simulink model "downlink_8c4t"  (Simulink 8.7)
settings: Solver=VariableStepDiscrete  StartTime=0.0  StopTime=20000  RelTol=1e-3
PreLoadFcn:
  | % Run the setup script when the model is opened
  | setup_downlink_8c4t;
InitFcn:
  | % Run the setup script again just before the
  | % model is run, so that any updates made
  | % after opening are applied.
  | 
  | setup_downlink_8c4t;
  | 
  | 
  | %% DSPBuilder Start
  | alt_dspbuilder_update_model(bdroot)
  | %% DSPBuilder End
values from neighbouring files (symbols this model uses):
  LUTS =     [downlink_8c4t_luts2.mat]
undefined symbols (not defined in the file or in its folder): DUC_LINEUP_param, value
libraries: DSPBAModelBus x44, DSPBABase x9, pipereg_lib x6, blind_cfr_lib x4, hduc_lib x4, dpd_lib x4, simulink x2, mixer_lib x2, lduc_lib x2, summer_4c4t_lib x2, DSPBAPrim x1
(part 1 of 2)
Description:
  | DSP Builder Advanced Template for Template Design implementing ModelIP designs
settings Model: Creator=mjervis  LastModifiedBy=5g
settings DataIOCC: SignalLoggingSaveFormat=ModelDataLogs
settings OptimizationCC: ExpressionDepthLimit=2147483647
settings DebuggingCC: SolverPrmCheckMsg=warning  InheritedTsInSrcMsg=none  IntegerOverflowMsg=none  FcnCallInpInsideContextMsg=UseLocalSettings  StateNameClashWarn=warning  IntegerSaturationMsg=none
settings GRTTargetCC: CombineOutputUpdateFcns=off  GRTInterface=on
settings ConfigComp: CovSFcnEnable=off

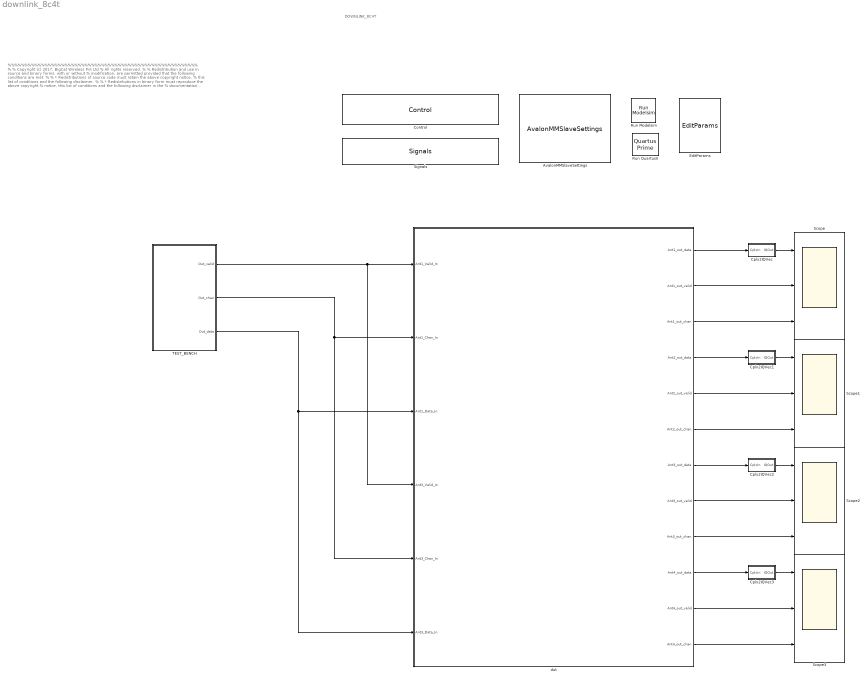
== system downlink_8c4t ==
  note: %%%%%%%%%%%%%%%%%%%%%%%%%%%%%%%%%%%%%%%%%%%%%%%%%%%%%%%%%
      | %
      | % Copyright (c) 2017, BigCat Wireless Pvt Ltd
      | % All rights reserved.
      | %
      | % Redistribution and use in source and binary forms, with or without
      | % modification, are permitted provided that the following conditions are met:
      | %
      | % * Redistributions of source code must retain the above copyright notice,
      | % this list of conditions and the following disclaimer.
      | %
      | % * Redistributions in binary form must reproduce the above copyright
      | % notice, this list of conditions and the following disclaimer in the
      | % documentation and/or other materials provided with the distribution.
      | %
      | % * Neither the name of the copyright holder nor the names of its contributors
      | % may be used to endorse or promote products derived from this software
      | % without specific prior written permission.
      | %
      | %
      | %
      | % THIS SOFTWARE IS PROVIDED BY THE COPYRIGHT HOLDERS AND CONTRIBUTORS "AS IS"
      | % AND ANY EXPRESS OR IMPLIED WARRANTIES, INCLUDING, BUT NOT LIMITED TO, THE
      | % IMPLIED WARRANTIES OF MERCHANTABILITY AND FITNESS FOR A PARTICULAR PURPOSE ARE
      | % DISCLAIMED. IN NO EVENT SHALL THE COPYRIGHT HOLDER OR CONTRIBUTORS BE LIABLE
      | % FOR ANY DIRECT, INDIRECT, INCIDENTAL, SPECIAL, EXEMPLARY, OR CONSEQUENTIAL
      | % DAMAGES (INCLUDING, BUT NOT LIMITED TO, PROCUREMENT OF SUBSTITUTE GOODS OR
      | % SERVICES; LOSS OF USE, DATA, OR PROFITS; OR BUSINESS INTERRUPTION) HOWEVER
      | % CAUSED AND ON ANY THEORY OF LIABILITY, WHETHER IN CONTRACT, STRICT LIABILITY,
      | % OR TORT (INCLUDING NEGLIGENCE OR OTHERWISE) ARISING IN ANY WAY OUT OF THE USE
      | % OF THIS SOFTWARE, EVEN IF ADVISED OF THE POSSIBILITY OF SUCH DAMAGE.
      | %
      | %%%%%%%%%%%%%%%%%%%%%%%%%%%%%%%%%%%%%%%%%%%%%%%%%%%%%%%%%%
  note: DOWNLINK_8C4T
  AvalonMMSlaveSettings : DSPBABase/AvalonMMSlaveSettings
  Control : DSPBABase/Control  generate=on  language=VHDL  destination=./rtl  destination_gui=./rtl  make_full_path=off  path_is_relative=on  autotestbench=off  signaldepth=2  coveragetestbench=off  logs=off  spacewidth=2  spacenum=1  addrwidth=13  datawidth=32  dataendian=Big Endian  hierarchicalnames=off  ramThresholdBits=-1  distRamThresholdBits=-1  mlabThresholdBits=-1  hardMultiplierThresholdLuts=-1  version=20090407  errorOnChanMismatch=1  errorOnGPIOMismatch=0  importModelsimResults=0  cycleAccurate=off  reinterpretCastMult=off  paramFile=downlink_8c4t_params.xml
  Cplx2IQVec : Subsystem
  Cplx2IQVec1 : Subsystem
  Cplx2IQVec2 : Subsystem
  Cplx2IQVec3 : Subsystem
  EditParams : DSPBABase/EditParams  version=20090407
  Run Modelsim : DSPBABase/Run Modelsim  version=20090407
  "Run QuartusII " : DSPBABase/Quartus Prime  version=20090407
  Scope{,1..3} (4 alike) : Scope  NumInputPorts=3
  Signals : DSPBABase/Signals  clk=clk  freq=DUC_LINEUP_param.ClockRate  margin=DUC_LINEUP_param.ClockMargin  rst=areset  rstactive=High  bus=bus  enbusclock=on  busfreq=61.44  bussync=on  version=20090407
  TEST_BENCH : Subsystem
  dut : Subsystem
  wires:
  TEST_BENCH/2(Out_chan) -> dut/5(Ant3_Chan_In), dut/2(Ant1_Chan_In)
  TEST_BENCH/3(Out_data) -> dut/6(Ant3_Data_In), dut/3(Ant1_Data_In)
  TEST_BENCH/1(Out_valid) -> dut/4(Ant3_Valid_In), dut/1(Ant1_Valid_In)
  dut/1(Ant1_out_data) -> Cplx2IQVec/1(CplxIn)
  dut/2(Ant1_out_valid) -> Scope/2
  dut/3(Ant1_out_chan) -> Scope/3
  dut/4(Ant2_out_data) -> Cplx2IQVec1/1(CplxIn)
  dut/5(Ant2_out_valid) -> Scope1/2
  dut/6(Ant2_out_chan) -> Scope1/3
  dut/7(Ant3_out_data) -> Cplx2IQVec2/1(CplxIn)
  dut/8(Ant3_out_valid) -> Scope2/2
  dut/9(Ant3_out_chan) -> Scope2/3
  dut/10(Ant4_out_data) -> Cplx2IQVec3/1(CplxIn)
  dut/11(Ant4_out_valid) -> Scope3/2
  dut/12(Ant4_out_chan) -> Scope3/3
  Cplx2IQVec/1(IQOut) -> Scope/1
  Cplx2IQVec1/1(IQOut) -> Scope1/1
  Cplx2IQVec2/1(IQOut) -> Scope2/1
  Cplx2IQVec3/1(IQOut) -> Scope3/1

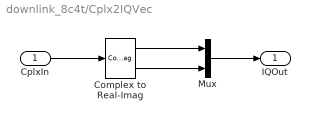
== system downlink_8c4t/Cplx2IQVec ==
  CplxIn : Inport
  Complex to Real-Imag : ComplexToRealImag
  Mux : Mux  Inputs=2
  IQOut : Outport
  wires:
  Complex to Real-Imag/1 -> Mux/1
  Mux/1 -> IQOut/1
  Complex to Real-Imag/2 -> Mux/2
  CplxIn/1 -> Complex to Real-Imag/1

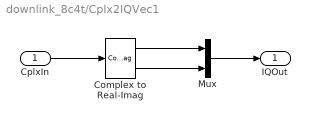
== system downlink_8c4t/Cplx2IQVec1 ==
  CplxIn : Inport
  Complex to Real-Imag : ComplexToRealImag
  Mux : Mux  Inputs=2
  IQOut : Outport
  wires:
  CplxIn/1 -> Complex to Real-Imag/1
  Complex to Real-Imag/2 -> Mux/2
  Mux/1 -> IQOut/1
  Complex to Real-Imag/1 -> Mux/1

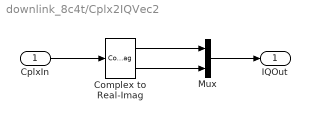
== system downlink_8c4t/Cplx2IQVec2 ==
  CplxIn : Inport
  Complex to Real-Imag : ComplexToRealImag
  Mux : Mux  Inputs=2
  IQOut : Outport
  wires:
  Complex to Real-Imag/1 -> Mux/1
  Mux/1 -> IQOut/1
  Complex to Real-Imag/2 -> Mux/2
  CplxIn/1 -> Complex to Real-Imag/1

== system downlink_8c4t/Cplx2IQVec3 ==
  CplxIn : Inport
  Complex to Real-Imag : ComplexToRealImag
  Mux : Mux  Inputs=2
  IQOut : Outport
  wires:
  CplxIn/1 -> Complex to Real-Imag/1
  Complex to Real-Imag/2 -> Mux/2
  Mux/1 -> IQOut/1
  Complex to Real-Imag/1 -> Mux/1

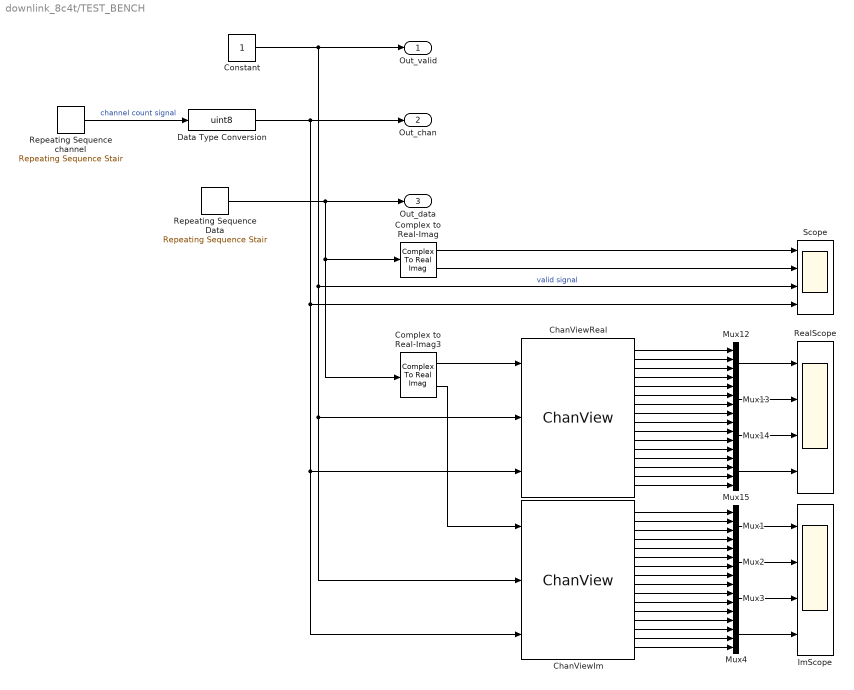
== system downlink_8c4t/TEST_BENCH ==
  ChanViewIm : DSPBABase/ChanView  nchans=16  chan_vector=[0:15]  outsvalid=off  latency=1  version=20090407
  ChanViewReal : DSPBABase/ChanView  nchans=16  chan_vector=[0:15]  outsvalid=off  latency=1  version=20090407
  Complex to Real-Imag : ComplexToRealImag
  Complex to Real-Imag3 : ComplexToRealImag
  Constant : Constant  OutDataTypeStr=boolean  SampleTime=1
  Data Type Conversion : DataTypeConversion  OutDataTypeStr=uint8
  ImScope : Scope  NumInputPorts=4
  Mux{1..4,12..15} (8 alike) : Mux
  RealScope : Scope  NumInputPorts=4
  Repeating Sequence Data : simulink/Sources/Repeating Sequence Stair  OutValues=DUC_LINEUP_param.inputdata  tsamp=1  OutMin=[]  OutMax=[]  OutDataTypeStr=fixdt(1,16,15)  OutputDataTypeScalingMode=Specify via dialog  OutDataType=fixdt(1,16,15)  ConRadixGroup=Best Precision: Vector-wise  OutScaling=[]
  Repeating Sequence channel : simulink/Sources/Repeating Sequence Stair  OutValues=[0:15].'  tsamp=1  OutMin=[]  OutMax=[]  OutDataTypeStr=uint8  OutputDataTypeScalingMode=uint8  OutDataType=fixdt(1,16)  ConRadixGroup=Best Precision: Vector-wise  OutScaling=[]
  Scope : Scope  NumInputPorts=4
  Out_valid : Outport
  Out_chan : Outport  Port=2
  Out_data : Outport  Port=3
  wires:
  Repeating Sequence Data/1 -> Out_data/1, Complex to Real-Imag/1, Complex to Real-Imag3/1
  Complex to Real-Imag/1 -> Scope/1
  Constant/1 -> Out_valid/1, ChanViewIm/2, ChanViewReal/2, Scope/3  "valid signal"
  Repeating Sequence channel/1 -> Data Type Conversion/1  "channel count signal"
  Complex to Real-Imag/2 -> Scope/2
  Mux12/1 -> RealScope/1
  Mux13/1 -> RealScope/2
  Mux14/1 -> RealScope/3
  Mux15/1 -> RealScope/4
  Complex to Real-Imag3/1 -> ChanViewReal/1
  Complex to Real-Imag3/2 -> ChanViewIm/1
  ChanViewReal/2 -> Mux12/2
  ChanViewReal/4 -> Mux12/4
  ChanViewReal/1 -> Mux12/1
  ChanViewReal/3 -> Mux12/3
  ChanViewReal/8 -> Mux13/4
  ChanViewReal/5 -> Mux13/1
  ChanViewReal/6 -> Mux13/2
  ChanViewReal/7 -> Mux13/3
  ChanViewReal/12 -> Mux14/4
  ChanViewReal/9 -> Mux14/1
  ChanViewReal/11 -> Mux14/3
  ChanViewReal/10 -> Mux14/2
  ChanViewReal/15 -> Mux15/3
  ChanViewReal/13 -> Mux15/1
  ChanViewReal/16 -> Mux15/4
  ChanViewReal/14 -> Mux15/2
  Mux1/1 -> ImScope/1
  Mux2/1 -> ImScope/2
  Mux3/1 -> ImScope/3
  Mux4/1 -> ImScope/4
  ChanViewIm/2 -> Mux1/2
  ChanViewIm/4 -> Mux1/4
  ChanViewIm/1 -> Mux1/1
  ChanViewIm/3 -> Mux1/3
  ChanViewIm/8 -> Mux2/4
  ChanViewIm/5 -> Mux2/1
  ChanViewIm/6 -> Mux2/2
  ChanViewIm/7 -> Mux2/3
  ChanViewIm/12 -> Mux3/4
  ChanViewIm/9 -> Mux3/1
  ChanViewIm/11 -> Mux3/3
  ChanViewIm/10 -> Mux3/2
  ChanViewIm/15 -> Mux4/3
  ChanViewIm/13 -> Mux4/1
  ChanViewIm/16 -> Mux4/4
  ChanViewIm/14 -> Mux4/2
  Data Type Conversion/1 -> Out_chan/1, ChanViewIm/3, ChanViewReal/3, Scope/4

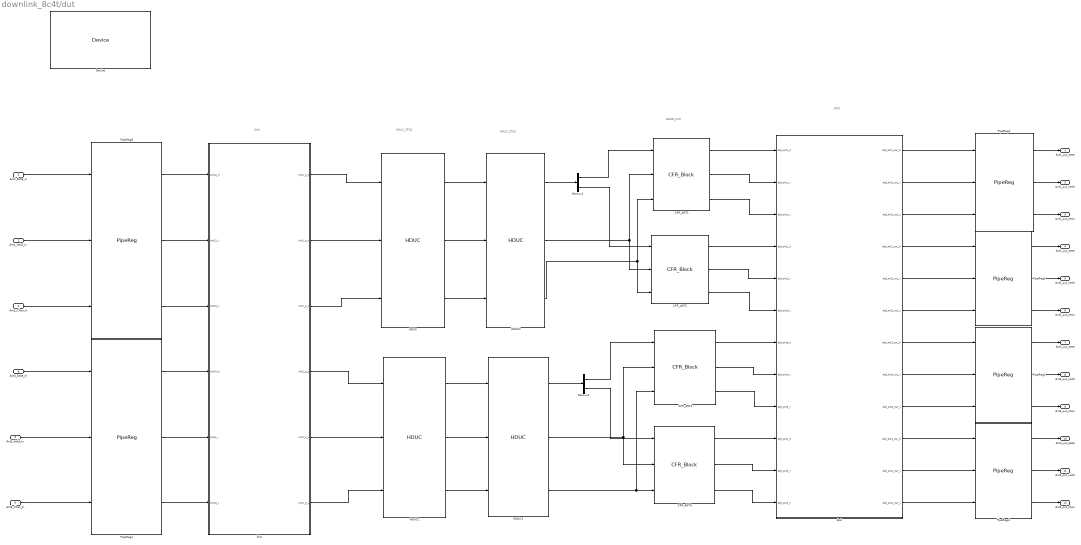
== system downlink_8c4t/dut ==
  note: DUC
  note: DPD
  note: BLIND_CFR
  note: HDUC_STG2
  note: HDUC_STG1
  Ant1_Valid_In : Inport
  Ant1_Chan_In : Inport  Port=2
  Ant1_Data_In : Inport  Port=3
  Ant3_Valid_In : Inport  Port=4
  Ant3_Chan_In : Inport  Port=5
  Ant3_Data_In : Inport  Port=6
  CFR_ANT1 : blind_cfr_lib/CFR_Block  clk=clock_rate  sample_rate=sample_rate  block_id=cfr0_id  block_id_addr=REG_dut_id_addr  cfr_Params=cfr_Params_Ant1  REG=REG  Pipeline_stages=0  ClockMargin=DUC_LINEUP_param.ClockMargin_CFR
      link override CFR/CPG gen/ChannelOut: latency=25
      link override CFR/PeakCan/ChannelOut1: latency=12
      link override CFR/PulseScale/ChannelOut: latency=25
      link override PipeReg/ChannelOut: latency=0
      link override PipeReg1/ChannelOut: latency=0
  CFR_ANT2 : blind_cfr_lib/CFR_Block  clk=clock_rate  sample_rate=sample_rate  block_id=cfr0_id  block_id_addr=REG_dut_id_addr  cfr_Params=cfr_Params_Ant2  REG=REG  Pipeline_stages=0  ClockMargin=DUC_LINEUP_param.ClockMargin_CFR
      link override CFR/CPG gen/ChannelOut: latency=25
      link override CFR/PeakCan/ChannelOut1: latency=12
      link override CFR/PulseScale/ChannelOut: latency=25
      link override PipeReg/ChannelOut: latency=0
      link override PipeReg1/ChannelOut: latency=0
  CFR_ANT3 : blind_cfr_lib/CFR_Block  clk=clock_rate  sample_rate=sample_rate  block_id=cfr0_id  block_id_addr=REG_dut_id_addr  cfr_Params=cfr_Params_Ant3  REG=REG  Pipeline_stages=0  ClockMargin=DUC_LINEUP_param.ClockMargin_CFR
      link override CFR/CPG gen/ChannelOut: latency=25
      link override CFR/PeakCan/ChannelOut1: latency=12
      link override CFR/PulseScale/ChannelOut: latency=25
      link override PipeReg/ChannelOut: latency=0
      link override PipeReg1/ChannelOut: latency=0
  CFR_ANT4 : blind_cfr_lib/CFR_Block  clk=clock_rate  sample_rate=sample_rate  block_id=cfr0_id  block_id_addr=REG_dut_id_addr  cfr_Params=cfr_Params_Ant4  REG=REG  Pipeline_stages=0  ClockMargin=DUC_LINEUP_param.ClockMargin_CFR
      link override CFR/CPG gen/ChannelOut: latency=25
      link override CFR/PeakCan/ChannelOut1: latency=12
      link override CFR/PulseScale/ChannelOut: latency=25
      link override PipeReg/ChannelOut: latency=0
      link override PipeReg1/ChannelOut: latency=0
  Demux1 : Demux  Outputs=2
  Demux4 : Demux  Outputs=2
  Device : DSPBABase/Device  family=Arria 10  deviceMember=Arria 10  stratix4device=Stratix IV GX  hardcopy4device=HardCopy IV E  stratix5device=Stratix V GX  device=10AS066N2F40I1SGES  speed=1  stratixSpeed=-5  stratix2Speed=-3  stratix3Speed=-3  stratix4gxSpeed=-2  stratix4gtSpeed=-1  cyclone2Speed=-6  cyclone3Speed=-7  arria2Speed=-4  cyclone4eSpeed=-8  stratix5Speed=-3  arria5Speed=-4  arriaSpeed=-6  cyclone3lsSpeed=-7  cyclone5Speed=-6  arria2gzSpeed=-3  nightFurySpeed=-2  ecp2Speed=-7  hardcopycompat=off  version=20140217  max10flashmode=off  max10nomeminit=off
  HDUC : hduc_lib/HDUC  HB_filt_SampleRate=DUC_LINEUP_param.HB_filt6.SampleRate  HB_filt_Interpolation=DUC_LINEUP_param.HB_filt6.Interpolation  HB_filt_ChanCount=DUC_LINEUP_param.HB_filt6.ChanCount  HB_filt_coeffs=DUC_LINEUP_param.HB_filt6.coeffs(1,:)  HB_filt_base_addr=DUC_LINEUP_param.HB_filt6.base_addr1  output_word_length=DUC_LINEUP_param.output_word_length  output_fraction_length=DUC_LINEUP_param.output_fraction_length  Multiplication_factor=DUC_LINEUP_param.HB_filt6.Mult_factor  Bits_to_shift_left=DUC_LINEUP_param.HB_filt6.left_shift  Pipeline_stages=2  ClockMargin=DUC_LINEUP_param.ClockMargin
      link override HB_filter: latency=14
      link override HB_filter1: latency=14
      link override scale_HB_filter: latency=6
      link override scale_HB_filter1: latency=6
  HDUC1 : hduc_lib/HDUC  HB_filt_SampleRate=DUC_LINEUP_param.HB_filt6.SampleRate  HB_filt_Interpolation=DUC_LINEUP_param.HB_filt6.Interpolation  HB_filt_ChanCount=DUC_LINEUP_param.HB_filt6.ChanCount  HB_filt_coeffs=DUC_LINEUP_param.HB_filt6.coeffs(1,:)  HB_filt_base_addr=DUC_LINEUP_param.HB_filt6.base_addr2  output_word_length=DUC_LINEUP_param.output_word_length  output_fraction_length=DUC_LINEUP_param.output_fraction_length  Multiplication_factor=DUC_LINEUP_param.HB_filt6.Mult_factor  Bits_to_shift_left=DUC_LINEUP_param.HB_filt6.left_shift  Pipeline_stages=2  ClockMargin=DUC_LINEUP_param.ClockMargin
      link override HB_filter: latency=14
      link override HB_filter1: latency=14
      link override scale_HB_filter: latency=6
      link override scale_HB_filter1: latency=6
  HDUC2 : hduc_lib/HDUC  HB_filt_SampleRate=DUC_LINEUP_param.HB_filt7.SampleRate  HB_filt_Interpolation=DUC_LINEUP_param.HB_filt7.Interpolation  HB_filt_ChanCount=DUC_LINEUP_param.HB_filt7.ChanCount  HB_filt_coeffs=DUC_LINEUP_param.HB_filt7.coeffs(1,:)  HB_filt_base_addr=DUC_LINEUP_param.HB_filt7.base_addr1  output_word_length=DUC_LINEUP_param.HB_filt7.coeff_word_length  output_fraction_length=DUC_LINEUP_param.HB_filt7.coeff_fraction_length  Multiplication_factor=DUC_LINEUP_param.HB_filt7.Mult_factor  Bits_to_shift_left=DUC_LINEUP_param.HB_filt7.left_shift  Pipeline_stages=2  ClockMargin=DUC_LINEUP_param.ClockMargin
      link override HB_filter: latency=7
      link override HB_filter1: latency=7
      link override scale_HB_filter: latency=6
      link override scale_HB_filter1: latency=6
  HDUC3 : hduc_lib/HDUC  HB_filt_SampleRate=DUC_LINEUP_param.HB_filt7.SampleRate  HB_filt_Interpolation=DUC_LINEUP_param.HB_filt7.Interpolation  HB_filt_ChanCount=DUC_LINEUP_param.HB_filt7.ChanCount  HB_filt_coeffs=DUC_LINEUP_param.HB_filt7.coeffs(1,:)  HB_filt_base_addr=DUC_LINEUP_param.HB_filt7.base_addr2  output_word_length=DUC_LINEUP_param.HB_filt7.coeff_word_length  output_fraction_length=DUC_LINEUP_param.HB_filt7.coeff_fraction_length  Multiplication_factor=DUC_LINEUP_param.HB_filt7.Mult_factor  Bits_to_shift_left=DUC_LINEUP_param.HB_filt7.left_shift  Pipeline_stages=0  ClockMargin=DUC_LINEUP_param.ClockMargin
      link override HB_filter: latency=7
      link override HB_filter1: latency=7
      link override scale_HB_filter: latency=6
      link override scale_HB_filter1: latency=6
  PipeReg1 : pipereg_lib/PipeReg  NPipe=6  Clock_Margin=DUC_LINEUP_param.ClockMargin
      link override ChannelOut: value=1  packetBeginEnabled=off  latency=6
  PipeReg2 : pipereg_lib/PipeReg  NPipe=6  Clock_Margin=DUC_LINEUP_param.ClockMargin
      link override ChannelOut: value=1  packetBeginEnabled=off  latency=6
  PipeReg3 : pipereg_lib/PipeReg  NPipe=6  Clock_Margin=DUC_LINEUP_param.ClockMargin
      link override ChannelOut: value=1  packetBeginEnabled=off  latency=6
  PipeReg4 : pipereg_lib/PipeReg  NPipe=6  Clock_Margin=DUC_LINEUP_param.ClockMargin
      link override ChannelOut: value=1  packetBeginEnabled=off  latency=6
  PipeReg6 : pipereg_lib/PipeReg  NPipe=6  Clock_Margin=DUC_LINEUP_param.ClockMargin
      link override ChannelOut: value=1  packetBeginEnabled=off  latency=6
  PipeReg8 : pipereg_lib/PipeReg  NPipe=6  Clock_Margin=DUC_LINEUP_param.ClockMargin
      link override ChannelOut: value=1  packetBeginEnabled=off  latency=6
  dpd : Subsystem
  lduc : Subsystem
  Ant1_out_data : Outport
  Ant1_out_valid : Outport  Port=2
  Ant1_out_chan : Outport  Port=3
  Ant2_out_data : Outport  Port=4
  Ant2_out_valid : Outport  Port=5
  Ant2_out_chan : Outport  Port=6
  Ant3_out_data : Outport  Port=7
  Ant3_out_valid : Outport  Port=8
  Ant3_out_chan : Outport  Port=9
  Ant4_out_data : Outport  Port=10
  Ant4_out_valid : Outport  Port=11
  Ant4_out_chan : Outport  Port=12
  wires:
  Ant1_Valid_In/1 -> PipeReg8/2
  Ant1_Chan_In/1 -> PipeReg8/3
  Ant3_Valid_In/1 -> PipeReg1/2
  Ant3_Chan_In/1 -> PipeReg1/3
  dpd/2(dpd_ant1_out_v) -> PipeReg2/2
  dpd/3(dpd_ant1_out_c) -> PipeReg2/3
  Ant1_Data_In/1 -> PipeReg8/1
  Ant3_Data_In/1 -> PipeReg1/1
  lduc/2(Ant1_q_v) -> HDUC/2
  lduc/5(Ant2_q_v) -> HDUC1/2
  lduc/6(Ant2_q_c) -> HDUC1/3
  HDUC/2 -> HDUC2/2
  HDUC/3 -> HDUC2/3
  HDUC/1 -> HDUC2/1
  HDUC1/2 -> HDUC3/2
  HDUC1/3 -> HDUC3/3
  HDUC1/1 -> HDUC3/1
  HDUC2/1 -> Demux1/1
  HDUC3/1 -> Demux4/1
  CFR_ANT1/2 -> dpd/2(dpd_ant1_v)
  CFR_ANT1/3 -> dpd/3(dpd_ant1_c)
  CFR_ANT2/1 -> dpd/4(dpd_ant2_d)
  CFR_ANT2/2 -> dpd/5(dpd_ant2_v)
  CFR_ANT2/3 -> dpd/6(dpd_ant2_c)
  CFR_ANT3/1 -> dpd/7(dpd_ant3_d)
  CFR_ANT3/2 -> dpd/8(dpd_ant3_v)
  CFR_ANT3/3 -> dpd/9(dpd_ant3_c)
  CFR_ANT4/1 -> dpd/10(dpd_ant4_d)
  CFR_ANT4/2 -> dpd/11(dpd_ant4_v)
  CFR_ANT4/3 -> dpd/12(dpd_ant4_c)
  PipeReg8/1 -> lduc/1(Ant12_d)
  PipeReg8/2 -> lduc/2(Ant12_v)
  PipeReg8/3 -> lduc/3(Ant12_c)
  PipeReg1/1 -> lduc/4(Ant34_d)
  PipeReg1/2 -> lduc/5(An34_v)
  PipeReg1/3 -> lduc/6(Ant34_c)
  lduc/1(Ant1_q_d) -> HDUC/1
  lduc/3(Ant1_q_c) -> HDUC/3
  lduc/4(Ant2_q_d) -> HDUC1/1
  Demux1/2 -> CFR_ANT2/1
  HDUC2/2 -> CFR_ANT2/2, CFR_ANT1/2
  HDUC2/3 -> CFR_ANT2/3, CFR_ANT1/3
  Demux4/1 -> CFR_ANT3/1
  HDUC3/2 -> CFR_ANT4/2, CFR_ANT3/2
  HDUC3/3 -> CFR_ANT4/3, CFR_ANT3/3
  Demux4/2 -> CFR_ANT4/1
  dpd/4(dpd_ant2_out_d) -> PipeReg6/1
  dpd/5(dpd_ant2_out_v) -> PipeReg6/2
  dpd/6(dpd_ant2_out_c) -> PipeReg6/3
  dpd/7(dpd_ant3_out_d) -> PipeReg3/1
  dpd/8(dpd_ant3_out_v) -> PipeReg3/2
  dpd/9(dpd_ant3_out_c) -> PipeReg3/3
  dpd/10(dpd_ant4_out_d) -> PipeReg4/1
  dpd/11(dpd_ant4_out_v) -> PipeReg4/2
  dpd/12(dpd_ant4_out_c) -> PipeReg4/3
  PipeReg2/1 -> Ant1_out_data/1
  PipeReg2/2 -> Ant1_out_valid/1
  PipeReg2/3 -> Ant1_out_chan/1
  PipeReg6/1 -> Ant2_out_data/1
  PipeReg6/2 -> Ant2_out_valid/1
  PipeReg6/3 -> Ant2_out_chan/1
  PipeReg3/1 -> Ant3_out_data/1
  PipeReg3/2 -> Ant3_out_valid/1
  PipeReg3/3 -> Ant3_out_chan/1
  PipeReg4/1 -> Ant4_out_data/1
  PipeReg4/2 -> Ant4_out_valid/1
  PipeReg4/3 -> Ant4_out_chan/1
  dpd/1(dpd_ant1_out_d) -> PipeReg2/1
  CFR_ANT1/1 -> dpd/1(dpd_ant1_d)
  Demux1/1 -> CFR_ANT1/1

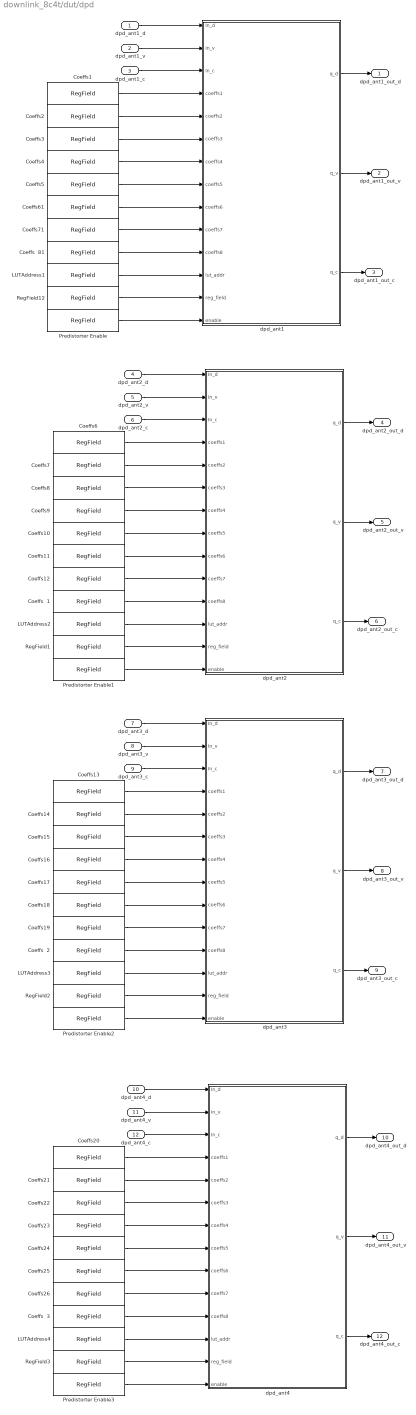
== system downlink_8c4t/dut/dpd ==
  dpd_ant1_d : Inport
  dpd_ant1_v : Inport  Port=2
  dpd_ant1_c : Inport  Port=3
  dpd_ant2_d : Inport  Port=4
  dpd_ant2_v : Inport  Port=5
  dpd_ant2_c : Inport  Port=6
  dpd_ant3_d : Inport  Port=7
  dpd_ant3_v : Inport  Port=8
  dpd_ant3_c : Inport  Port=9
  dpd_ant4_d : Inport  Port=10
  dpd_ant4_v : Inport  Port=11
  dpd_ant4_c : Inport  Port=12
  Coeffs  1 : DSPBAModelBus/RegField  reg_name=dpd2_StartAddress10  reg_rwmode=Read/Write  reg_msb=2*(DUC_LINEUP_param.input_word_length)-1  reg_lsb=0  reg_mode=Specify via dialog  reg_type=ufix(2*DUC_LINEUP_param.input_word_length)  reg_scale=1  reg_init=0  reg_desc=I and Q coeffs for the next LUT entrance  reg_modal=off  reg_desc0=0  reg_desc1=0  reg_desc2=0  reg_desc3=0  reg_desc4=0  reg_desc5=0  reg_desc6=0  reg_desc7=0  reg_addr=9050  SampleTime=-1  version=20090407
  Coeffs  2 : DSPBAModelBus/RegField  reg_name=dpd3_StartAddress10  reg_rwmode=Read/Write  reg_msb=2*(DUC_LINEUP_param.input_word_length)-1  reg_lsb=0  reg_mode=Specify via dialog  reg_type=ufix(2*DUC_LINEUP_param.input_word_length)  reg_scale=1  reg_init=0  reg_desc=I and Q coeffs for the next LUT entrance  reg_modal=off  reg_desc0=0  reg_desc1=0  reg_desc2=0  reg_desc3=0  reg_desc4=0  reg_desc5=0  reg_desc6=0  reg_desc7=0  reg_addr=9062  SampleTime=-1  version=20090407
  Coeffs  3 : DSPBAModelBus/RegField  reg_name=dpd4_StartAddress10  reg_rwmode=Read/Write  reg_msb=2*(DUC_LINEUP_param.input_word_length)-1  reg_lsb=0  reg_mode=Specify via dialog  reg_type=ufix(2*DUC_LINEUP_param.input_word_length)  reg_scale=1  reg_init=0  reg_desc=I and Q coeffs for the next LUT entrance  reg_modal=off  reg_desc0=0  reg_desc1=0  reg_desc2=0  reg_desc3=0  reg_desc4=0  reg_desc5=0  reg_desc6=0  reg_desc7=0  reg_addr=9074  SampleTime=-1  version=20090407
  Coeffs  81 : DSPBAModelBus/RegField  reg_name=dpd1_StartAddress10  reg_rwmode=Read/Write  reg_msb=2*(DUC_LINEUP_param.input_word_length)-1  reg_lsb=0  reg_mode=Specify via dialog  reg_type=ufix(2*DUC_LINEUP_param.input_word_length)  reg_scale=1  reg_init=0  reg_desc=I and Q coeffs for the next LUT entrance  reg_modal=off  reg_desc0=0  reg_desc1=0  reg_desc2=0  reg_desc3=0  reg_desc4=0  reg_desc5=0  reg_desc6=0  reg_desc7=0  reg_addr=9038  SampleTime=-1  version=20090407
  Coeffs1 : DSPBAModelBus/RegField  reg_name=dpd1_StartAddress3  reg_rwmode=Read/Write  reg_msb=2*(DUC_LINEUP_param.input_word_length)-1  reg_lsb=0  reg_mode=Specify via dialog  reg_type=ufix(2*DUC_LINEUP_param.input_word_length)  reg_scale=1  reg_init=0  reg_desc=I and Q coeffs for the next LUT entrance  reg_modal=off  reg_desc0=0  reg_desc1=0  reg_desc2=0  reg_desc3=0  reg_desc4=0  reg_desc5=0  reg_desc6=0  reg_desc7=0  reg_addr=9031  SampleTime=-1  version=20090407
  Coeffs10 : DSPBAModelBus/RegField  reg_name=dpd2_StartAddress7  reg_rwmode=Read/Write  reg_msb=2*(DUC_LINEUP_param.input_word_length)-1  reg_lsb=0  reg_mode=Specify via dialog  reg_type=ufix(2*DUC_LINEUP_param.input_word_length)  reg_scale=1  reg_init=0  reg_desc=I and Q coeffs for the next LUT entrance  reg_modal=off  reg_desc0=0  reg_desc1=0  reg_desc2=0  reg_desc3=0  reg_desc4=0  reg_desc5=0  reg_desc6=0  reg_desc7=0  reg_addr=9047  SampleTime=-1  version=20090407
  Coeffs11 : DSPBAModelBus/RegField  reg_name=dpd2_StartAddress8  reg_rwmode=Read/Write  reg_msb=2*(DUC_LINEUP_param.input_word_length)-1  reg_lsb=0  reg_mode=Specify via dialog  reg_type=ufix(2*DUC_LINEUP_param.input_word_length)  reg_scale=1  reg_init=0  reg_desc=I and Q coeffs for the next LUT entrance  reg_modal=off  reg_desc0=0  reg_desc1=0  reg_desc2=0  reg_desc3=0  reg_desc4=0  reg_desc5=0  reg_desc6=0  reg_desc7=0  reg_addr=9048  SampleTime=-1  version=20090407
  Coeffs12 : DSPBAModelBus/RegField  reg_name=dpd2_StartAddress9  reg_rwmode=Read/Write  reg_msb=2*(DUC_LINEUP_param.input_word_length)-1  reg_lsb=0  reg_mode=Specify via dialog  reg_type=ufix(2*DUC_LINEUP_param.input_word_length)  reg_scale=1  reg_init=0  reg_desc=I and Q coeffs for the next LUT entrance  reg_modal=off  reg_desc0=0  reg_desc1=0  reg_desc2=0  reg_desc3=0  reg_desc4=0  reg_desc5=0  reg_desc6=0  reg_desc7=0  reg_addr=9049  SampleTime=-1  version=20090407
  Coeffs13 : DSPBAModelBus/RegField  reg_name=dpd3_StartAddress3  reg_rwmode=Read/Write  reg_msb=2*(DUC_LINEUP_param.input_word_length)-1  reg_lsb=0  reg_mode=Specify via dialog  reg_type=ufix(2*DUC_LINEUP_param.input_word_length)  reg_scale=1  reg_init=0  reg_desc=I and Q coeffs for the next LUT entrance  reg_modal=off  reg_desc0=0  reg_desc1=0  reg_desc2=0  reg_desc3=0  reg_desc4=0  reg_desc5=0  reg_desc6=0  reg_desc7=0  reg_addr=9055  SampleTime=-1  version=20090407
  Coeffs14 : DSPBAModelBus/RegField  reg_name=dpd3_StartAddress4  reg_rwmode=Read/Write  reg_msb=2*(DUC_LINEUP_param.input_word_length)-1  reg_lsb=0  reg_mode=Specify via dialog  reg_type=ufix(2*DUC_LINEUP_param.input_word_length)  reg_scale=1  reg_init=0  reg_desc=I and Q coeffs for the next LUT entrance  reg_modal=off  reg_desc0=0  reg_desc1=0  reg_desc2=0  reg_desc3=0  reg_desc4=0  reg_desc5=0  reg_desc6=0  reg_desc7=0  reg_addr=9056  SampleTime=-1  version=20090407
  Coeffs15 : DSPBAModelBus/RegField  reg_name=dpd3_StartAddress5  reg_rwmode=Read/Write  reg_msb=2*(DUC_LINEUP_param.input_word_length)-1  reg_lsb=0  reg_mode=Specify via dialog  reg_type=ufix(2*DUC_LINEUP_param.input_word_length)  reg_scale=1  reg_init=0  reg_desc=I and Q coeffs for the next LUT entrance  reg_modal=off  reg_desc0=0  reg_desc1=0  reg_desc2=0  reg_desc3=0  reg_desc4=0  reg_desc5=0  reg_desc6=0  reg_desc7=0  reg_addr=9057  SampleTime=-1  version=20090407
  Coeffs16 : DSPBAModelBus/RegField  reg_name=dpd3_StartAddress6  reg_rwmode=Read/Write  reg_msb=2*(DUC_LINEUP_param.input_word_length)-1  reg_lsb=0  reg_mode=Specify via dialog  reg_type=ufix(2*DUC_LINEUP_param.input_word_length)  reg_scale=1  reg_init=0  reg_desc=I and Q coeffs for the next LUT entrance  reg_modal=off  reg_desc0=0  reg_desc1=0  reg_desc2=0  reg_desc3=0  reg_desc4=0  reg_desc5=0  reg_desc6=0  reg_desc7=0  reg_addr=9058  SampleTime=-1  version=20090407
  Coeffs17 : DSPBAModelBus/RegField  reg_name=dpd3_StartAddress7  reg_rwmode=Read/Write  reg_msb=2*(DUC_LINEUP_param.input_word_length)-1  reg_lsb=0  reg_mode=Specify via dialog  reg_type=ufix(2*DUC_LINEUP_param.input_word_length)  reg_scale=1  reg_init=0  reg_desc=I and Q coeffs for the next LUT entrance  reg_modal=off  reg_desc0=0  reg_desc1=0  reg_desc2=0  reg_desc3=0  reg_desc4=0  reg_desc5=0  reg_desc6=0  reg_desc7=0  reg_addr=9059  SampleTime=-1  version=20090407
  Coeffs18 : DSPBAModelBus/RegField  reg_name=dpd3_StartAddress8  reg_rwmode=Read/Write  reg_msb=2*(DUC_LINEUP_param.input_word_length)-1  reg_lsb=0  reg_mode=Specify via dialog  reg_type=ufix(2*DUC_LINEUP_param.input_word_length)  reg_scale=1  reg_init=0  reg_desc=I and Q coeffs for the next LUT entrance  reg_modal=off  reg_desc0=0  reg_desc1=0  reg_desc2=0  reg_desc3=0  reg_desc4=0  reg_desc5=0  reg_desc6=0  reg_desc7=0  reg_addr=9060  SampleTime=-1  version=20090407
  Coeffs19 : DSPBAModelBus/RegField  reg_name=dpd3_StartAddress9  reg_rwmode=Read/Write  reg_msb=2*(DUC_LINEUP_param.input_word_length)-1  reg_lsb=0  reg_mode=Specify via dialog  reg_type=ufix(2*DUC_LINEUP_param.input_word_length)  reg_scale=1  reg_init=0  reg_desc=I and Q coeffs for the next LUT entrance  reg_modal=off  reg_desc0=0  reg_desc1=0  reg_desc2=0  reg_desc3=0  reg_desc4=0  reg_desc5=0  reg_desc6=0  reg_desc7=0  reg_addr=9061  SampleTime=-1  version=20090407
  Coeffs2 : DSPBAModelBus/RegField  reg_name=dpd1_StartAddress4  reg_rwmode=Read/Write  reg_msb=2*(DUC_LINEUP_param.input_word_length)-1  reg_lsb=0  reg_mode=Specify via dialog  reg_type=ufix(2*DUC_LINEUP_param.input_word_length)  reg_scale=1  reg_init=0  reg_desc=I and Q coeffs for the next LUT entrance  reg_modal=off  reg_desc0=0  reg_desc1=0  reg_desc2=0  reg_desc3=0  reg_desc4=0  reg_desc5=0  reg_desc6=0  reg_desc7=0  reg_addr=9032  SampleTime=-1  version=20090407
  Coeffs20 : DSPBAModelBus/RegField  reg_name=dpd4_StartAddress3  reg_rwmode=Read/Write  reg_msb=2*(DUC_LINEUP_param.input_word_length)-1  reg_lsb=0  reg_mode=Specify via dialog  reg_type=ufix(2*DUC_LINEUP_param.input_word_length)  reg_scale=1  reg_init=0  reg_desc=I and Q coeffs for the next LUT entrance  reg_modal=off  reg_desc0=0  reg_desc1=0  reg_desc2=0  reg_desc3=0  reg_desc4=0  reg_desc5=0  reg_desc6=0  reg_desc7=0  reg_addr=9067  SampleTime=-1  version=20090407
  Coeffs21 : DSPBAModelBus/RegField  reg_name=dpd4_StartAddress4  reg_rwmode=Read/Write  reg_msb=2*(DUC_LINEUP_param.input_word_length)-1  reg_lsb=0  reg_mode=Specify via dialog  reg_type=ufix(2*DUC_LINEUP_param.input_word_length)  reg_scale=1  reg_init=0  reg_desc=I and Q coeffs for the next LUT entrance  reg_modal=off  reg_desc0=0  reg_desc1=0  reg_desc2=0  reg_desc3=0  reg_desc4=0  reg_desc5=0  reg_desc6=0  reg_desc7=0  reg_addr=9068  SampleTime=-1  version=20090407
  Coeffs22 : DSPBAModelBus/RegField  reg_name=dpd4_StartAddress5  reg_rwmode=Read/Write  reg_msb=2*(DUC_LINEUP_param.input_word_length)-1  reg_lsb=0  reg_mode=Specify via dialog  reg_type=ufix(2*DUC_LINEUP_param.input_word_length)  reg_scale=1  reg_init=0  reg_desc=I and Q coeffs for the next LUT entrance  reg_modal=off  reg_desc0=0  reg_desc1=0  reg_desc2=0  reg_desc3=0  reg_desc4=0  reg_desc5=0  reg_desc6=0  reg_desc7=0  reg_addr=9069  SampleTime=-1  version=20090407
  Coeffs23 : DSPBAModelBus/RegField  reg_name=dpd4_StartAddress6  reg_rwmode=Read/Write  reg_msb=2*(DUC_LINEUP_param.input_word_length)-1  reg_lsb=0  reg_mode=Specify via dialog  reg_type=ufix(2*DUC_LINEUP_param.input_word_length)  reg_scale=1  reg_init=0  reg_desc=I and Q coeffs for the next LUT entrance  reg_modal=off  reg_desc0=0  reg_desc1=0  reg_desc2=0  reg_desc3=0  reg_desc4=0  reg_desc5=0  reg_desc6=0  reg_desc7=0  reg_addr=9070  SampleTime=-1  version=20090407
  Coeffs24 : DSPBAModelBus/RegField  reg_name=dpd4_StartAddress7  reg_rwmode=Read/Write  reg_msb=2*(DUC_LINEUP_param.input_word_length)-1  reg_lsb=0  reg_mode=Specify via dialog  reg_type=ufix(2*DUC_LINEUP_param.input_word_length)  reg_scale=1  reg_init=0  reg_desc=I and Q coeffs for the next LUT entrance  reg_modal=off  reg_desc0=0  reg_desc1=0  reg_desc2=0  reg_desc3=0  reg_desc4=0  reg_desc5=0  reg_desc6=0  reg_desc7=0  reg_addr=9071  SampleTime=-1  version=20090407
  Coeffs25 : DSPBAModelBus/RegField  reg_name=dpd4_StartAddress8  reg_rwmode=Read/Write  reg_msb=2*(DUC_LINEUP_param.input_word_length)-1  reg_lsb=0  reg_mode=Specify via dialog  reg_type=ufix(2*DUC_LINEUP_param.input_word_length)  reg_scale=1  reg_init=0  reg_desc=I and Q coeffs for the next LUT entrance  reg_modal=off  reg_desc0=0  reg_desc1=0  reg_desc2=0  reg_desc3=0  reg_desc4=0  reg_desc5=0  reg_desc6=0  reg_desc7=0  reg_addr=9072  SampleTime=-1  version=20090407
  Coeffs26 : DSPBAModelBus/RegField  reg_name=dpd4_StartAddress9  reg_rwmode=Read/Write  reg_msb=2*(DUC_LINEUP_param.input_word_length)-1  reg_lsb=0  reg_mode=Specify via dialog  reg_type=ufix(2*DUC_LINEUP_param.input_word_length)  reg_scale=1  reg_init=0  reg_desc=I and Q coeffs for the next LUT entrance  reg_modal=off  reg_desc0=0  reg_desc1=0  reg_desc2=0  reg_desc3=0  reg_desc4=0  reg_desc5=0  reg_desc6=0  reg_desc7=0  reg_addr=9073  SampleTime=-1  version=20090407
  Coeffs3 : DSPBAModelBus/RegField  reg_name=dpd1_StartAddress5  reg_rwmode=Read/Write  reg_msb=2*(DUC_LINEUP_param.input_word_length)-1  reg_lsb=0  reg_mode=Specify via dialog  reg_type=ufix(2*DUC_LINEUP_param.input_word_length)  reg_scale=1  reg_init=0  reg_desc=I and Q coeffs for the next LUT entrance  reg_modal=off  reg_desc0=0  reg_desc1=0  reg_desc2=0  reg_desc3=0  reg_desc4=0  reg_desc5=0  reg_desc6=0  reg_desc7=0  reg_addr=9033  SampleTime=-1  version=20090407
  Coeffs4 : DSPBAModelBus/RegField  reg_name=dpd1_StartAddress6  reg_rwmode=Read/Write  reg_msb=2*(DUC_LINEUP_param.input_word_length)-1  reg_lsb=0  reg_mode=Specify via dialog  reg_type=ufix(2*DUC_LINEUP_param.input_word_length)  reg_scale=1  reg_init=0  reg_desc=I and Q coeffs for the next LUT entrance  reg_modal=off  reg_desc0=0  reg_desc1=0  reg_desc2=0  reg_desc3=0  reg_desc4=0  reg_desc5=0  reg_desc6=0  reg_desc7=0  reg_addr=9034  SampleTime=-1  version=20090407
  Coeffs5 : DSPBAModelBus/RegField  reg_name=dpd1_StartAddress7  reg_rwmode=Read/Write  reg_msb=2*(DUC_LINEUP_param.input_word_length)-1  reg_lsb=0  reg_mode=Specify via dialog  reg_type=ufix(2*DUC_LINEUP_param.input_word_length)  reg_scale=1  reg_init=0  reg_desc=I and Q coeffs for the next LUT entrance  reg_modal=off  reg_desc0=0  reg_desc1=0  reg_desc2=0  reg_desc3=0  reg_desc4=0  reg_desc5=0  reg_desc6=0  reg_desc7=0  reg_addr=9035  SampleTime=-1  version=20090407
  Coeffs6 : DSPBAModelBus/RegField  reg_name=dpd2_StartAddress3  reg_rwmode=Read/Write  reg_msb=2*(DUC_LINEUP_param.input_word_length)-1  reg_lsb=0  reg_mode=Specify via dialog  reg_type=ufix(2*DUC_LINEUP_param.input_word_length)  reg_scale=1  reg_init=0  reg_desc=I and Q coeffs for the next LUT entrance  reg_modal=off  reg_desc0=0  reg_desc1=0  reg_desc2=0  reg_desc3=0  reg_desc4=0  reg_desc5=0  reg_desc6=0  reg_desc7=0  reg_addr=9043  SampleTime=-1  version=20090407
  Coeffs61 : DSPBAModelBus/RegField  reg_name=dpd1_StartAddress8  reg_rwmode=Read/Write  reg_msb=2*(DUC_LINEUP_param.input_word_length)-1  reg_lsb=0  reg_mode=Specify via dialog  reg_type=ufix(2*DUC_LINEUP_param.input_word_length)  reg_scale=1  reg_init=0  reg_desc=I and Q coeffs for the next LUT entrance  reg_modal=off  reg_desc0=0  reg_desc1=0  reg_desc2=0  reg_desc3=0  reg_desc4=0  reg_desc5=0  reg_desc6=0  reg_desc7=0  reg_addr=9036  SampleTime=-1  version=20090407
  Coeffs7 : DSPBAModelBus/RegField  reg_name=dpd2_StartAddress4  reg_rwmode=Read/Write  reg_msb=2*(DUC_LINEUP_param.input_word_length)-1  reg_lsb=0  reg_mode=Specify via dialog  reg_type=ufix(2*DUC_LINEUP_param.input_word_length)  reg_scale=1  reg_init=0  reg_desc=I and Q coeffs for the next LUT entrance  reg_modal=off  reg_desc0=0  reg_desc1=0  reg_desc2=0  reg_desc3=0  reg_desc4=0  reg_desc5=0  reg_desc6=0  reg_desc7=0  reg_addr=9044  SampleTime=-1  version=20090407
  Coeffs71 : DSPBAModelBus/RegField  reg_name=dpd1_StartAddress9  reg_rwmode=Read/Write  reg_msb=2*(DUC_LINEUP_param.input_word_length)-1  reg_lsb=0  reg_mode=Specify via dialog  reg_type=ufix(2*DUC_LINEUP_param.input_word_length)  reg_scale=1  reg_init=0  reg_desc=I and Q coeffs for the next LUT entrance  reg_modal=off  reg_desc0=0  reg_desc1=0  reg_desc2=0  reg_desc3=0  reg_desc4=0  reg_desc5=0  reg_desc6=0  reg_desc7=0  reg_addr=9037  SampleTime=-1  version=20090407
  Coeffs8 : DSPBAModelBus/RegField  reg_name=dpd2_StartAddress5  reg_rwmode=Read/Write  reg_msb=2*(DUC_LINEUP_param.input_word_length)-1  reg_lsb=0  reg_mode=Specify via dialog  reg_type=ufix(2*DUC_LINEUP_param.input_word_length)  reg_scale=1  reg_init=0  reg_desc=I and Q coeffs for the next LUT entrance  reg_modal=off  reg_desc0=0  reg_desc1=0  reg_desc2=0  reg_desc3=0  reg_desc4=0  reg_desc5=0  reg_desc6=0  reg_desc7=0  reg_addr=9045  SampleTime=-1  version=20090407
  Coeffs9 : DSPBAModelBus/RegField  reg_name=dpd2_StartAddress6  reg_rwmode=Read/Write  reg_msb=2*(DUC_LINEUP_param.input_word_length)-1  reg_lsb=0  reg_mode=Specify via dialog  reg_type=ufix(2*DUC_LINEUP_param.input_word_length)  reg_scale=1  reg_init=0  reg_desc=I and Q coeffs for the next LUT entrance  reg_modal=off  reg_desc0=0  reg_desc1=0  reg_desc2=0  reg_desc3=0  reg_desc4=0  reg_desc5=0  reg_desc6=0  reg_desc7=0  reg_addr=9046  SampleTime=-1  version=20090407
  LUTAddress1 : DSPBAModelBus/RegField  reg_name=dpd1_StartAddress2  reg_rwmode=Read/Write  reg_msb=ceil(log2(size(LUTS.ENTRIES,1)))  reg_lsb=0  reg_mode=Specify via dialog  reg_type=ufix(log2(size(LUTS.ENTRIES,1)) + 1)  reg_scale=1  reg_init=0  reg_desc=LUT address for Coeff update  reg_modal=off  reg_desc0=0  reg_desc1=0  reg_desc2=0  reg_desc3=0  reg_desc4=0  reg_desc5=0  reg_desc6=0  reg_desc7=0  reg_addr=9030  SampleTime=-1  version=20090407
  LUTAddress2 : DSPBAModelBus/RegField  reg_name=dpd2_StartAddress2  reg_rwmode=Read/Write  reg_msb=ceil(log2(size(LUTS.ENTRIES,1)))  reg_lsb=0  reg_mode=Specify via dialog  reg_type=ufix(log2(size(LUTS.ENTRIES,1)) + 1)  reg_scale=1  reg_init=0  reg_desc=LUT address for Coeff update  reg_modal=off  reg_desc0=0  reg_desc1=0  reg_desc2=0  reg_desc3=0  reg_desc4=0  reg_desc5=0  reg_desc6=0  reg_desc7=0  reg_addr=9042  SampleTime=-1  version=20090407
  LUTAddress3 : DSPBAModelBus/RegField  reg_name=dpd3_StartAddress2  reg_rwmode=Read/Write  reg_msb=ceil(log2(size(LUTS.ENTRIES,1)))  reg_lsb=0  reg_mode=Specify via dialog  reg_type=ufix(log2(size(LUTS.ENTRIES,1)) + 1)  reg_scale=1  reg_init=0  reg_desc=LUT address for Coeff update  reg_modal=off  reg_desc0=0  reg_desc1=0  reg_desc2=0  reg_desc3=0  reg_desc4=0  reg_desc5=0  reg_desc6=0  reg_desc7=0  reg_addr=9054  SampleTime=-1  version=20090407
  LUTAddress4 : DSPBAModelBus/RegField  reg_name=dpd4_StartAddress2  reg_rwmode=Read/Write  reg_msb=ceil(log2(size(LUTS.ENTRIES,1)))  reg_lsb=0  reg_mode=Specify via dialog  reg_type=ufix(log2(size(LUTS.ENTRIES,1)) + 1)  reg_scale=1  reg_init=0  reg_desc=LUT address for Coeff update  reg_modal=off  reg_desc0=0  reg_desc1=0  reg_desc2=0  reg_desc3=0  reg_desc4=0  reg_desc5=0  reg_desc6=0  reg_desc7=0  reg_addr=9066  SampleTime=-1  version=20090407
  Predistorter Enable : DSPBAModelBus/RegField  reg_name=dpd1_StartAddress12  reg_rwmode=Read/Write  reg_msb=0  reg_lsb=0  reg_mode=Specify via dialog  reg_type=ufix(1)  reg_scale=2^0  reg_init=1  reg_desc=Enable the DPD  reg_modal=off  reg_desc0=0  reg_desc1=0  reg_desc2=0  reg_desc3=0  reg_desc4=0  reg_desc5=0  reg_desc6=0  reg_desc7=0  reg_addr=9040  SampleTime=-1  version=20090407
  Predistorter Enable1 : DSPBAModelBus/RegField  reg_name=dpd2_StartAddress12  reg_rwmode=Read/Write  reg_msb=0  reg_lsb=0  reg_mode=Specify via dialog  reg_type=ufix(1)  reg_scale=2^0  reg_init=1  reg_desc=Enable the DPD  reg_modal=off  reg_desc0=0  reg_desc1=0  reg_desc2=0  reg_desc3=0  reg_desc4=0  reg_desc5=0  reg_desc6=0  reg_desc7=0  reg_addr=9052  SampleTime=-1  version=20090407
  Predistorter Enable2 : DSPBAModelBus/RegField  reg_name=dpd3_StartAddress12  reg_rwmode=Read/Write  reg_msb=0  reg_lsb=0  reg_mode=Specify via dialog  reg_type=ufix(1)  reg_scale=2^0  reg_init=1  reg_desc=Enable the DPD  reg_modal=off  reg_desc0=0  reg_desc1=0  reg_desc2=0  reg_desc3=0  reg_desc4=0  reg_desc5=0  reg_desc6=0  reg_desc7=0  reg_addr=9064  SampleTime=-1  version=20090407
  Predistorter Enable3 : DSPBAModelBus/RegField  reg_name=dpd4_StartAddress12  reg_rwmode=Read/Write  reg_msb=0  reg_lsb=0  reg_mode=Specify via dialog  reg_type=ufix(1)  reg_scale=2^0  reg_init=1  reg_desc=Enable the DPD  reg_modal=off  reg_desc0=0  reg_desc1=0  reg_desc2=0  reg_desc3=0  reg_desc4=0  reg_desc5=0  reg_desc6=0  reg_desc7=0  reg_addr=9076  SampleTime=-1  version=20090407
  RegField1 : DSPBAModelBus/RegField  reg_name=dpd2_StartAddress11  reg_rwmode=Read/Write  reg_msb=0  reg_lsb=0  reg_mode=Specify via dialog  reg_type=ufix(1)  reg_scale=1  reg_init=0  reg_desc=Selects LUT bank  reg_modal=off  reg_desc0=0  reg_desc1=0  reg_desc2=0  reg_desc3=0  reg_desc4=0  reg_desc5=0  reg_desc6=0  reg_desc7=0  reg_addr=9051  SampleTime=-1  version=20090407
  RegField12 : DSPBAModelBus/RegField  reg_name=dpd1_StartAddress11  reg_rwmode=Read/Write  reg_msb=0  reg_lsb=0  reg_mode=Specify via dialog  reg_type=ufix(1)  reg_scale=1  reg_init=0  reg_desc=Selects LUT bank  reg_modal=off  reg_desc0=0  reg_desc1=0  reg_desc2=0  reg_desc3=0  reg_desc4=0  reg_desc5=0  reg_desc6=0  reg_desc7=0  reg_addr=9039  SampleTime=-1  version=20090407
  RegField2 : DSPBAModelBus/RegField  reg_name=dpd3_StartAddress11  reg_rwmode=Read/Write  reg_msb=0  reg_lsb=0  reg_mode=Specify via dialog  reg_type=ufix(1)  reg_scale=1  reg_init=0  reg_desc=Selects LUT bank  reg_modal=off  reg_desc0=0  reg_desc1=0  reg_desc2=0  reg_desc3=0  reg_desc4=0  reg_desc5=0  reg_desc6=0  reg_desc7=0  reg_addr=9063  SampleTime=-1  version=20090407
  RegField3 : DSPBAModelBus/RegField  reg_name=dpd4_StartAddress11  reg_rwmode=Read/Write  reg_msb=0  reg_lsb=0  reg_mode=Specify via dialog  reg_type=ufix(1)  reg_scale=1  reg_init=0  reg_desc=Selects LUT bank  reg_modal=off  reg_desc0=0  reg_desc1=0  reg_desc2=0  reg_desc3=0  reg_desc4=0  reg_desc5=0  reg_desc6=0  reg_desc7=0  reg_addr=9075  SampleTime=-1  version=20090407
  dpd_ant1 : Subsystem
  dpd_ant2 : Subsystem
  dpd_ant3 : Subsystem
  dpd_ant4 : Subsystem
  dpd_ant1_out_d : Outport
  dpd_ant1_out_v : Outport  Port=2
  dpd_ant1_out_c : Outport  Port=3
  dpd_ant2_out_d : Outport  Port=4
  dpd_ant2_out_v : Outport  Port=5
  dpd_ant2_out_c : Outport  Port=6
  dpd_ant3_out_d : Outport  Port=7
  dpd_ant3_out_v : Outport  Port=8
  dpd_ant3_out_c : Outport  Port=9
  dpd_ant4_out_d : Outport  Port=10
  dpd_ant4_out_v : Outport  Port=11
  dpd_ant4_out_c : Outport  Port=12
  wires:
  dpd_ant1/1(q_d) -> dpd_ant1_out_d/1
  dpd_ant1/2(q_v) -> dpd_ant1_out_v/1
  dpd_ant1/3(q_c) -> dpd_ant1_out_c/1
  dpd_ant1_d/1 -> dpd_ant1/1(In_d)
  dpd_ant1_v/1 -> dpd_ant1/2(In_v)
  dpd_ant1_c/1 -> dpd_ant1/3(In_c)
  dpd_ant2/1(q_d) -> dpd_ant2_out_d/1
  dpd_ant2/2(q_v) -> dpd_ant2_out_v/1
  dpd_ant2/3(q_c) -> dpd_ant2_out_c/1
  dpd_ant2_d/1 -> dpd_ant2/1(In_d)
  dpd_ant2_v/1 -> dpd_ant2/2(In_v)
  dpd_ant2_c/1 -> dpd_ant2/3(In_c)
  dpd_ant3/1(q_d) -> dpd_ant3_out_d/1
  dpd_ant3/2(q_v) -> dpd_ant3_out_v/1
  dpd_ant3/3(q_c) -> dpd_ant3_out_c/1
  dpd_ant3_d/1 -> dpd_ant3/1(In_d)
  dpd_ant3_v/1 -> dpd_ant3/2(In_v)
  dpd_ant3_c/1 -> dpd_ant3/3(In_c)
  dpd_ant4/1(q_d) -> dpd_ant4_out_d/1
  dpd_ant4/2(q_v) -> dpd_ant4_out_v/1
  dpd_ant4/3(q_c) -> dpd_ant4_out_c/1
  dpd_ant4_d/1 -> dpd_ant4/1(In_d)
  dpd_ant4_v/1 -> dpd_ant4/2(In_v)
  dpd_ant4_c/1 -> dpd_ant4/3(In_c)
  Coeffs1/1 -> dpd_ant1/4(coeffs1)
  Coeffs2/1 -> dpd_ant1/5(coeffs2)
  Coeffs3/1 -> dpd_ant1/6(coeffs3)
  Coeffs4/1 -> dpd_ant1/7(coeffs4)
  Coeffs5/1 -> dpd_ant1/8(coeffs5)
  Coeffs61/1 -> dpd_ant1/9(coeffs6)
  Coeffs71/1 -> dpd_ant1/10(coeffs7)
  Coeffs  81/1 -> dpd_ant1/11(coeffs8)
  LUTAddress1/1 -> dpd_ant1/12(lut_addr)
  Predistorter Enable/1 -> dpd_ant1/14(enable)
  RegField12/1 -> dpd_ant1/13(reg_field)
  Coeffs6/1 -> dpd_ant2/4(coeffs1)
  Coeffs7/1 -> dpd_ant2/5(coeffs2)
  Coeffs8/1 -> dpd_ant2/6(coeffs3)
  Coeffs9/1 -> dpd_ant2/7(coeffs4)
  Coeffs10/1 -> dpd_ant2/8(coeffs5)
  Coeffs11/1 -> dpd_ant2/9(coeffs6)
  Coeffs12/1 -> dpd_ant2/10(coeffs7)
  Coeffs  1/1 -> dpd_ant2/11(coeffs8)
  LUTAddress2/1 -> dpd_ant2/12(lut_addr)
  Predistorter Enable1/1 -> dpd_ant2/14(enable)
  RegField1/1 -> dpd_ant2/13(reg_field)
  Coeffs13/1 -> dpd_ant3/4(coeffs1)
  Coeffs14/1 -> dpd_ant3/5(coeffs2)
  Coeffs15/1 -> dpd_ant3/6(coeffs3)
  Coeffs16/1 -> dpd_ant3/7(coeffs4)
  Coeffs17/1 -> dpd_ant3/8(coeffs5)
  Coeffs18/1 -> dpd_ant3/9(coeffs6)
  Coeffs19/1 -> dpd_ant3/10(coeffs7)
  Coeffs  2/1 -> dpd_ant3/11(coeffs8)
  LUTAddress3/1 -> dpd_ant3/12(lut_addr)
  Predistorter Enable2/1 -> dpd_ant3/14(enable)
  RegField2/1 -> dpd_ant3/13(reg_field)
  Coeffs20/1 -> dpd_ant4/4(coeffs1)
  Coeffs21/1 -> dpd_ant4/5(coeffs2)
  Coeffs22/1 -> dpd_ant4/6(coeffs3)
  Coeffs23/1 -> dpd_ant4/7(coeffs4)
  Coeffs24/1 -> dpd_ant4/8(coeffs5)
  Coeffs25/1 -> dpd_ant4/9(coeffs6)
  Coeffs26/1 -> dpd_ant4/10(coeffs7)
  Coeffs  3/1 -> dpd_ant4/11(coeffs8)
  LUTAddress4/1 -> dpd_ant4/12(lut_addr)
  Predistorter Enable3/1 -> dpd_ant4/14(enable)
  RegField3/1 -> dpd_ant4/13(reg_field)
